simulink model "ex7"  (R2025b)
settings: Solver=VariableStepAuto  StartTime=0.0  StopTime=10.0  RelTol=1e-3
settings Model: Creator=vladl  LastModifiedBy=vladl

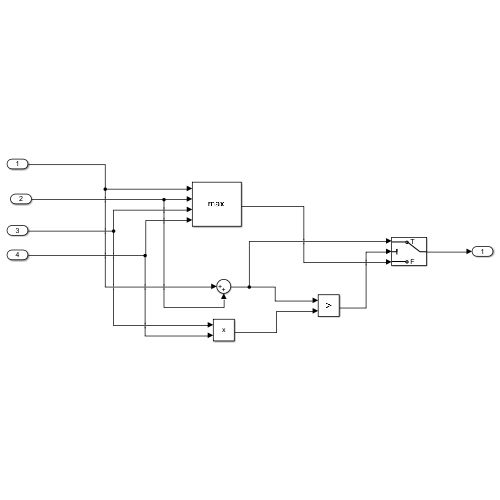
[thumbnail: Simulink's stored preview of the top-level diagram]
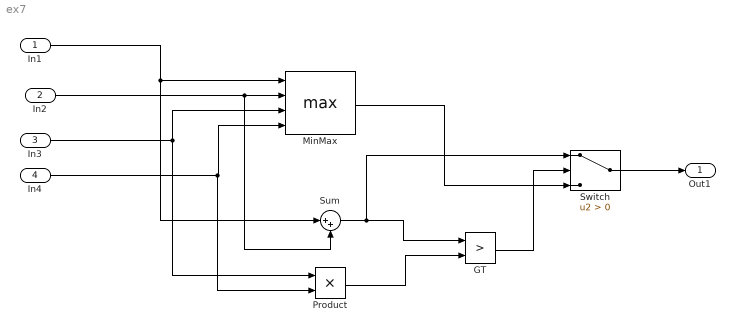
== system ex7 ==
  In1 : Inport
  In2 : Inport  Port=2
  In3 : Inport  Port=3
  In4 : Inport  Port=4
  GT : RelationalOperator  Operator=>  OutDataTypeStr=boolean  RndMeth=Simplest  InputSameDT=off
  MinMax : MinMax  Function=max  Inputs=4
  Product : Product
  Sum : Sum  Inputs=|++
  Switch : Switch  Criteria=u2 > Threshold  SaturateOnIntegerOverflow=off  InputSameDT=off
  Out1 : Outport
  wires:
  In1/1 -> Sum/1, MinMax/1
  In2/1 -> Sum/2, MinMax/2
  In3/1 -> MinMax/3, Product/1
  In4/1 -> Product/2, MinMax/4
  Sum/1 -> Switch/1, GT/1
  Product/1 -> GT/2
  GT/1 -> Switch/2
  MinMax/1 -> Switch/3
  Switch/1 -> Out1/1
